simulink subsystem "State_Estimation_2WD_NO_FILTER_NO_REGEN"  (R2023b)
settings: Solver=VariableStepAuto  StartTime=0.0  StopTime=10.0  RelTol=1e-3
settings Model: Creator=Inver  LastModifiedBy=Inver

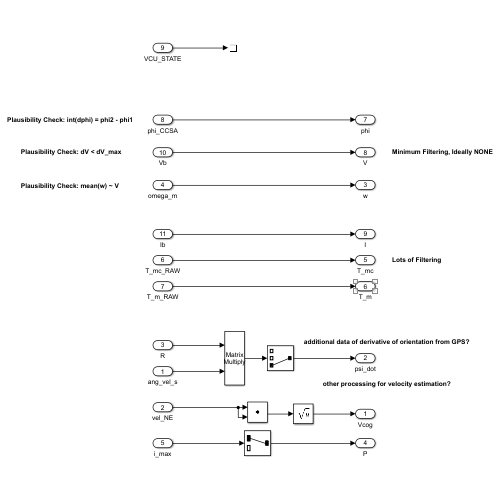
[thumbnail: Simulink's stored preview of the top-level diagram]
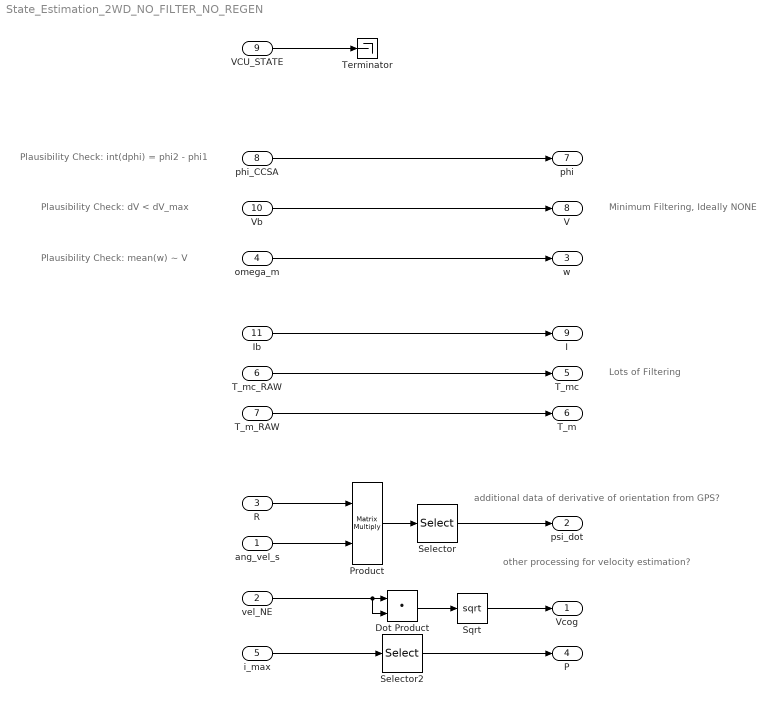
== system State_Estimation_2WD_NO_FILTER_NO_REGEN ==
  note: other processing for velocity estimation?
  note: additional data of derivative of orientation from GPS?
  note: Minimum Filtering, Ideally NONE
  note: Lots of Filtering
  note: Plausibility Check: int(dphi) = phi2 - phi1
  note: Plausibility Check: mean(w) ~ V
  note: Plausibility Check: dV < dV_max
  ang_vel_s : Inport
  vel_NE : Inport  Port=2
  R : Inport  Port=3
  omega_m : Inport  Port=4
  i_max : Inport  Port=5
  T_mc_RAW : Inport  Port=6
  T_m_RAW : Inport  Port=7
  phi_CCSA : Inport  Port=8
  VCU_STATE : Inport  Port=9
  Vb : Inport  Port=10
  Ib : Inport  Port=11
  Dot Product : DotProduct  OutDataTypeStr=Inherit: Inherit via internal rule
  Product : Product  Multiplication=Matrix(*)
  Selector : Selector  InputPortWidth=3  IndexOptions=Index vector (dialog)  Indices=[3]  OutputSizes=1
  Selector2 : Selector  InputPortWidth=2  IndexOptions=Index vector (dialog)  Indices=1  OutputSizes=1
  Sqrt : Sqrt
  Terminator : Terminator
  Vcog : Outport
  psi_dot : Outport  Port=2
  w : Outport  Port=3
  P : Outport  Port=4
  T_mc : Outport  Port=5
  T_m : Outport  Port=6
  phi : Outport  Port=7
  V : Outport  Port=8
  I : Outport  Port=9
  wires:
  ang_vel_s/1 -> Product/2
  R/1 -> Product/1
  Product/1 -> Selector/1
  Selector/1 -> psi_dot/1
  Dot Product/1 -> Sqrt/1
  vel_NE/1 -> Dot Product/2, Dot Product/1
  Sqrt/1 -> Vcog/1
  omega_m/1 -> w/1
  i_max/1 -> Selector2/1
  phi_CCSA/1 -> phi/1
  Vb/1 -> V/1
  VCU_STATE/1 -> Terminator/1
  Selector2/1 -> P/1
  Ib/1 -> I/1
  T_m_RAW/1 -> T_m/1
  T_mc_RAW/1 -> T_mc/1
